simulink model "robot_payload"  (R2021b)
settings: Solver=VariableStepAuto  StartTime=0.0  StopTime=76  RelTol=1e-3
libraries: roblocks x17, simulink x6
settings Model: Creator=sam  LastModifiedBy=sam

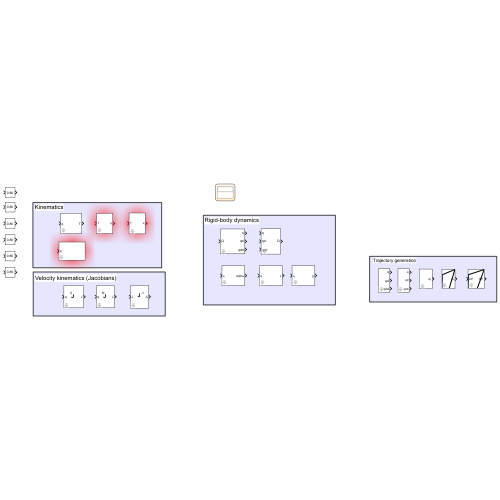
[thumbnail: Simulink's stored preview of the top-level diagram]
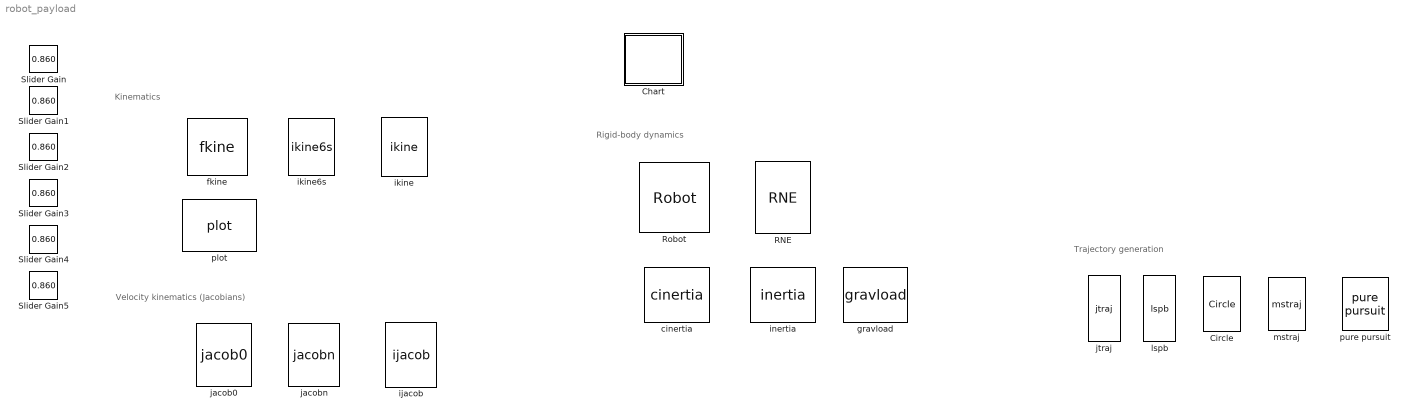
== system robot_payload ==
  note: Rigid-body dynamics
  note: Velocity kinematics (Jacobians)
  note: Kinematics
  note: Trajectory generation
  Chart : Stateflow chart  TreatAsAtomicUnit=on
  Circle : roblocks/Toolbox/Circle  radius=1  freq=0.2
  RNE : roblocks/Arm/RNE  robot=robot  grav=[0 0 9.81]
  Robot : roblocks/Arm/Robot  robot=robot  q0=[0 0 0 0 0 0]
  Slider Gain{,1..5} (6 alike) : simulink/Math Operations/Slider Gain  gain=0.860  low=0  high=2
  cinertia : roblocks/Arm/cinertia  robot=0
  fkine : roblocks/Arm/fkine  robot=robot
  gravload : roblocks/Arm/gravload  robot=0
  ijacob : roblocks/Arm/ijacob
  ikine : roblocks/Arm/ikine  robot=p560  q0=qz  M=[1 1 1 1 1 1]  pinv=off  options={}
  ikine6s : roblocks/Arm/ikine6s  robot=p560  conf='luf'
  inertia : roblocks/Arm/inertia  robot=0
  "jacob0 " : roblocks/Arm/jacob0   robot=robot
  jacobn : roblocks/Arm/jacobn  robot=robot
  jtraj : roblocks/Toolbox/jtraj  q0=[0 0 0 0 0 0]  qf=[pi/4 pi/2 -pi/2 0 0 0]  tmax=10  ts=0.02
  lspb : roblocks/Toolbox/lspb  q0=0  qf=0  tmax=0
  mstraj : roblocks/Toolbox/mstraj  path=|  vaxis=[2.5 2.5]  tseg=[]  dt=0.1  tacc=0  setsimtime=on
      | [  10 10;
      |   10 60;
      |   80 80;
      |   50 10 ]
  plot : roblocks/Arm/plot  robot=p560  fps=5  holdplot=on
  pure pursuit : roblocks/Toolbox/pure pursuit  path=|  vaxis=[2.5 2.5]  tseg=[]  dt=0.1  tacc=0  R=5
      | [  10 10;
      |   10 60;
      |   80 80;
      |   50 10 ]

== matlab function robot_payload/Chart ==
function
